simulink model "exer_2_2_3"  (R2014b)
settings: Solver=ode45  StartTime=0.0  StopTime=10.0  RelTol=1e-3
libraries: simulink x2, dspsnks4 x1
settings Model: Creator=Charlie  LastModifiedBy=Charlie

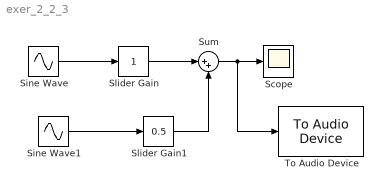
== system exer_2_2_3 ==
  Scope : Scope
  Sine Wave : Sin  Frequency=1000  SampleTime=1/48000
  Sine Wave1 : Sin  Frequency=2000  SampleTime=1/48000
  Slider Gain : simulink/Math Operations/Slider Gain  low=0  gain=1  high=2
  Slider Gain1 : simulink/Math Operations/Slider Gain  low=0  gain=0.5  high=2
  Sum : Sum  Inputs=|++
  To Audio Device : dspsnks4/To Audio Device  deviceName=Default  inheritSampleRate=on  sampleRate=44100  deviceDatatype=Determine from input data type  autoBufferSize=on  bufferSize=4096  queueDuration=1.0  defaultOutputChannelMapping=on  outputChannelMapping=1:2  outputNumUnderrunSamples=off
  wires:
  Sine Wave/1 -> Slider Gain/1
  Sine Wave1/1 -> Slider Gain1/1
  Sum/1 -> To Audio Device/1, Scope/1
  Slider Gain/1 -> Sum/1
  Slider Gain1/1 -> Sum/2
